simulink model "Day1"  (R2017b)
settings: Solver=VariableStepAuto  StartTime=0.0  StopTime=10.0  RelTol=1e-3
libraries: simulink x3
settings Model: Creator=Admin  LastModifiedBy=Admin

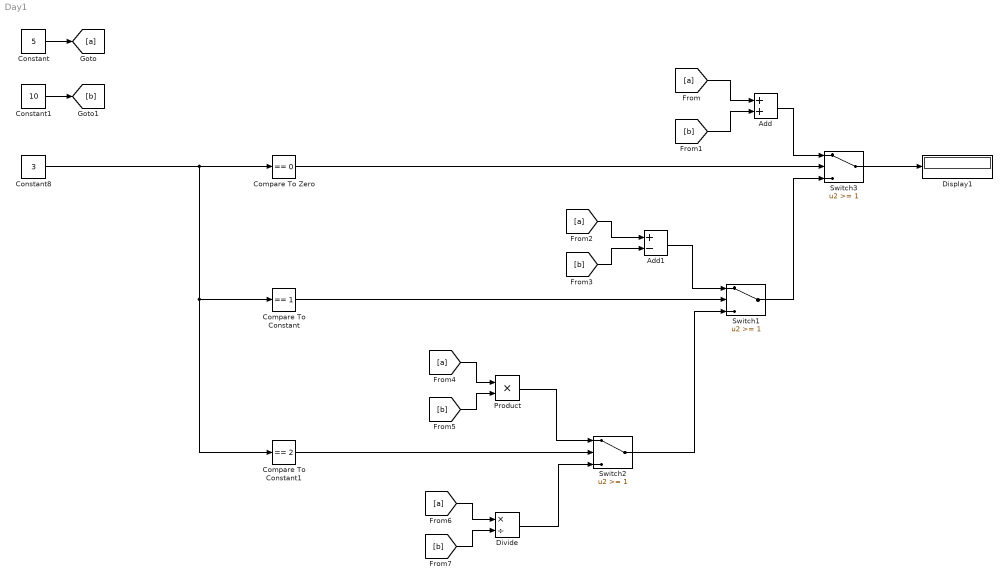
== system Day1 ==
  Add : Sum
  Add1 : Sum  Inputs=+-
  Compare To Constant : simulink/Logic and Bit Operations/Compare To Constant  relop===  const=1  OutDataTypeStr=boolean
  Compare To Constant1 : simulink/Logic and Bit Operations/Compare To Constant  relop===  const=2  OutDataTypeStr=boolean
  Compare To Zero : simulink/Logic and Bit Operations/Compare To Zero  relop===  OutDataTypeStr=boolean
  Constant : Constant  Value=5  OutDataTypeStr=double
  Constant1 : Constant  Value=10  OutDataTypeStr=double
  Constant8 : Constant  Value=3
  Display1 : Display
  Divide : Product  Inputs=*/
  Product : Product
  Switch1 : Switch  Threshold=1
  Switch2 : Switch  Threshold=1
  Switch3 : Switch  Threshold=1
  wires:
  [a] -> Add1/1
  [b] -> Add1/2
  [a] -> Product/1
  [b] -> Product/2
  [b] -> Divide/2
  [a] -> Divide/1
  Add/1 -> Switch3/1
  Switch3/1 -> Display1/1
  Switch1/1 -> Switch3/3
  Add1/1 -> Switch1/1
  Constant8/1 -> Compare To Zero/1, Compare To Constant1/1, Compare To Constant/1
  Switch2/1 -> Switch1/3
  Product/1 -> Switch2/1
  Constant/1 -> [a]
  [a] -> Add/1
  Constant1/1 -> [b]
  [b] -> Add/2
  Divide/1 -> Switch2/3
  Compare To Zero/1 -> Switch3/2
  Compare To Constant/1 -> Switch1/2
  Compare To Constant1/1 -> Switch2/2
